simulink model "SkywalkerX8_Control"  (R2018a)
settings: Solver=FixedStepAuto  StartTime=0.0  StopTime=120  FixedStep=0.01  RelTol=1e-3
undefined symbols (not defined in the file): sigbuilder_block, SkywalkerX8
libraries: simulink x5, simulink_extras x3
(part 1 of 2)
settings Model: Creator=David  LastModifiedBy=David
settings OptimizationCC: DefaultParameterBehavior=Inlined  EnhancedBackFolding=on  PassReuseOutputArgsThreshold=0  OptimizeBlockOrder=speed  DifferentSizesBufferReuse=on  OptimizationCustomize=off
settings DebuggingCC: ParameterTunabilityLossMsg=error
settings SFSimCC: MATLABDynamicMemAlloc=off
settings RTWCC: GenCodeOnly=on  Description=Generic Real-Time Target  GenerateReport=on  LaunchReport=on
settings CodeAppCC: ForceParamTrailComments=on  OperatorAnnotations=on

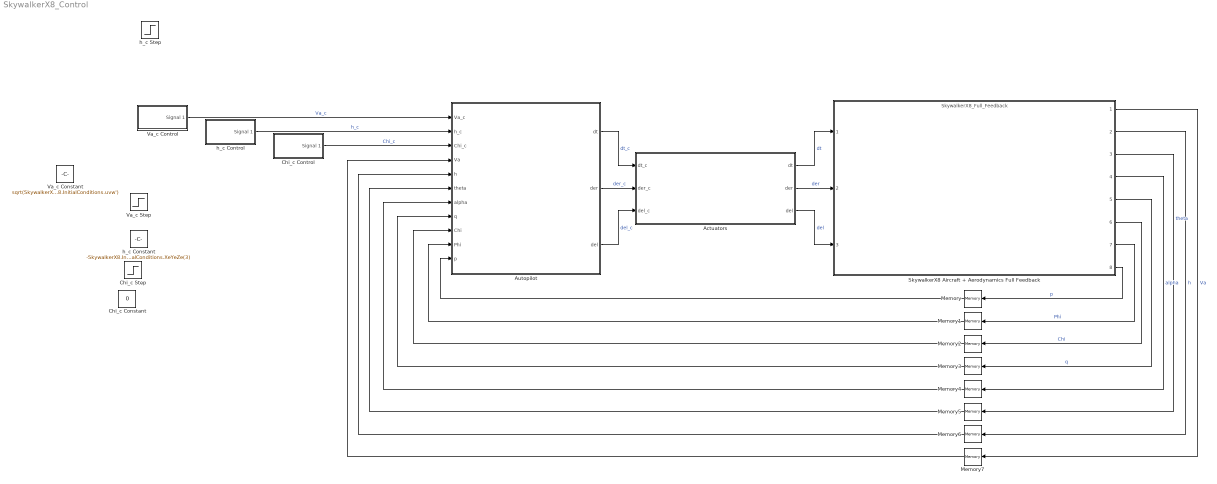
== system SkywalkerX8_Control ==
  Actuators : Subsystem
      mask Display:
      | image('actuators.jpg', 'center')
      | 
      | color('white')
      | 
      | port_label('input', 1, 'd_{t_c} (Unitless)', 'texmode', 'on')
      | port_label('input', 2, 'd_{{er}_c} (rad)', 'texmode', 'on')
      | port_label('input', 3, 'd_{{el}_c} (rad)', 'texmode', 'on')
      | 
      | port_label('output', 1, 'd_t (Unitless)', 'texmode', 'on')
      | port_label('output', 2, 'd_{er} (rad)', 'texmode', 'on')
      | port_label('output', 3, 'd_{el} (rad)', 'texmode', 'on')
  Autopilot : Subsystem
      mask Display:
      | image('autopilot.png', 'center')
      | 
      | port_label('output', 1, '\delta_t (Unitless)', 'texmode', 'on')
      | port_label('output', 2, '\delta_e_r (rad)', 'texmode', 'on')
      | port_label('output', 3, '\delta_e_l (rad)', 'texmode', 'on')
      | 
      | port_label('input', 1, 'V_{a_c} (m/s)', 'texmode', 'on')
      | port_label('input', 2, 'h_c (m)', 'texmode', 'on')
      | port_label('input', 3, '\chi_c (rad)', 'texmode', 'on')
      | port_label('input', 4, 'V_a (m/s)', 'texmode', 'on')
      | port_label('input', 5, 'Altitude (m)', 'texmode', 'on')
      | port_label('input', 6, '\theta (rad)', 'texmode', 'on')
      | port_label('input', 7, '\alpha (rad)', 'texmode', 'on')
      | port_label('input', 8, 'q (rad/s)', 'texmode', 'on')
      | port_label('input', 9, '\chi (rad)', 'texmode', 'on')
      | port_label('input', 10, '\phi (rad)', 'texmode', 'on')
      | port_label('input', 11, 'p (rad/s)', 'texmode', 'on')
  Chi_c Constant : Constant  Value=0
  Chi_c Control : Subsystem  Tag=STV Subsys  LoadFcn=sigbuilder_block('load');  StartFcn=sigbuilder_block('start');  StopFcn=sigbuilder_block('stop');  ClipboardFcn=sigbuilder_block('clipboard');  mask(Sigbuilder block){tuvar=[0:10]}
      mask help: Simulink:masks:SigbuilderBlock_MD
      mask init:
      | if ~strcmp(get_param(bdroot(gcbh),'SimulationStatus'),'stopped') tuvar = sigbuilder_block('maskInit'); end
      settings: CopyFcn=sigbuilder_block('copy');  DeleteFcn=sigbuilder_block('delete');  ModelCloseFcn=sigbuilder_block('modelClose');  PreSaveFcn=sigbuilder_block('preSave');  PauseFcn=sigbuilder_block('pause');  ContinueFcn=sigbuilder_block('continue');  NameChangeFcn=sigbuilder_block('namechange');  OpenFcn=sigbuilder_block('open',[437.6 199.2 550.4 400 ]);  CloseFcn=sigbuilder_block('close');
      mask Display: plot(0, 0, 100, 100,[2, 2, 32, 32, 2], [68, 8, 8, 68, 68],[32, 2], [38, 38], [32, 19, 2],[53, 60, 44], [32, 17, 17, 2],[16, 16, 31, 31]);txt = getActiveGroup(gcbh);text(2, 100, txt,'verticalAlignment', 'top');
  Chi_c Step : Step  After=deg2rad(90)  SampleTime=0
  Memory : Memory  InitialCondition=SkywalkerX8.InitialConditions.pqr(1)
  Memory1 : Memory  InitialCondition=SkywalkerX8.InitialConditions.PhiThetaPsi(1)
  Memory2 : Memory  InitialCondition=SkywalkerX8.InitialConditions.PhiThetaPsi(3)
  Memory3 : Memory  InitialCondition=SkywalkerX8.InitialConditions.pqr(2)
  Memory4 : Memory  InitialCondition=atan2(SkywalkerX8.InitialConditions.uvw(3), SkywalkerX8.InitialConditions.uvw(1))
  Memory5 : Memory  InitialCondition=SkywalkerX8.InitialConditions.PhiThetaPsi(2)
  Memory6 : Memory  InitialCondition=-SkywalkerX8.InitialConditions.XeYeZe(3)
  Memory7 : Memory  InitialCondition=sqrt(SkywalkerX8.InitialConditions.uvw*SkywalkerX8.InitialConditions.uvw')
  SkywalkerX8 Aircraft + Aerodynamics Full Feedback : ModelReference  ModelNameDialog=SkywalkerX8_Full_Feedback  ModelReferenceVersion=1.29
      mask Display:
      | image('x8SkySunset.png', 'center')
      | 
      | port_label('input', 1, '\delta_t (Unitless)', 'texmode', 'on')
      | port_label('input', 2, '\delta_e_r (rad)', 'texmode', 'on')
      | port_label('input', 3, '\delta_e_l (rad)', 'texmode', 'on')
      | 
      | port_label('output', 1, 'V_a (m/s)', 'texmode', 'on')
      | port_label('output', 2, 'Altitude (m)', 'texmode', 'on')
      | port_label('output', 3, '\theta (rad)', 'texmode', 'on')
      | port_label('output', 4, '\alpha (rad)', 'texmode', 'on')
      | port_label('output', 5, 'q (rad/s)', 'texmode', 'on')
      | port_label('output', 6, '\chi (rad)', 'texmode', 'on')
      | port_label('output', 7, '\phi (rad)', 'texmode', 'on')
      | port_label('output', 8, 'p (rad/s)', 'texmode', 'on')
  Va_c Constant : Constant  Value=sqrt(SkywalkerX8.InitialConditions.uvw*SkywalkerX8.InitialConditions.uvw')
  Va_c Control : Subsystem  Tag=STV Subsys  LoadFcn=sigbuilder_block('load');  StartFcn=sigbuilder_block('start');  StopFcn=sigbuilder_block('stop');  ClipboardFcn=sigbuilder_block('clipboard');  mask(Sigbuilder block){tuvar=[0:10]}
      mask help: Simulink:masks:SigbuilderBlock_MD
      mask init:
      | if ~strcmp(get_param(bdroot(gcbh),'SimulationStatus'),'stopped') tuvar = sigbuilder_block('maskInit'); end
      settings: CopyFcn=sigbuilder_block('copy');  DeleteFcn=sigbuilder_block('delete');  ModelCloseFcn=sigbuilder_block('modelClose');  PreSaveFcn=sigbuilder_block('preSave');  PauseFcn=sigbuilder_block('pause');  ContinueFcn=sigbuilder_block('continue');  NameChangeFcn=sigbuilder_block('namechange');  OpenFcn=sigbuilder_block('open',[437.6 199.2 550.4 400 ]);  CloseFcn=sigbuilder_block('close');
      mask Display: plot(0, 0, 100, 100,[2, 2, 32, 32, 2], [68, 8, 8, 68, 68],[32, 2], [38, 38], [32, 19, 2],[53, 60, 44], [32, 17, 17, 2],[16, 16, 31, 31]);txt = getActiveGroup(gcbh);text(2, 100, txt,'verticalAlignment', 'top');
  Va_c Step : Step  Before=sqrt(SkywalkerX8.InitialConditions.uvw*SkywalkerX8.InitialConditions.uvw')  After=sqrt(SkywalkerX8.InitialConditions.uvw*SkywalkerX8.InitialConditions.uvw')  SampleTime=0
  h_c Constant : Constant  Value=-SkywalkerX8.InitialConditions.XeYeZe(3)
  h_c Control : Subsystem  Tag=STV Subsys  LoadFcn=sigbuilder_block('load');  StartFcn=sigbuilder_block('start');  StopFcn=sigbuilder_block('stop');  ClipboardFcn=sigbuilder_block('clipboard');  mask(Sigbuilder block){tuvar=[0:10]}
      mask help: Simulink:masks:SigbuilderBlock_MD
      mask init:
      | if ~strcmp(get_param(bdroot(gcbh),'SimulationStatus'),'stopped') tuvar = sigbuilder_block('maskInit'); end
      settings: CopyFcn=sigbuilder_block('copy');  DeleteFcn=sigbuilder_block('delete');  ModelCloseFcn=sigbuilder_block('modelClose');  PreSaveFcn=sigbuilder_block('preSave');  PauseFcn=sigbuilder_block('pause');  ContinueFcn=sigbuilder_block('continue');  NameChangeFcn=sigbuilder_block('namechange');  OpenFcn=sigbuilder_block('open',[6 30 1428 771.75 ]);  CloseFcn=sigbuilder_block('close');
      mask Display: plot(0, 0, 100, 100,[2, 2, 32, 32, 2], [68, 8, 8, 68, 68],[32, 2], [38, 38], [32, 19, 2],[53, 60, 44], [32, 17, 17, 2],[16, 16, 31, 31]);txt = getActiveGroup(gcbh);text(2, 100, txt,'verticalAlignment', 'top');
  h_c Step : Step  Time=0.1  Before=-SkywalkerX8.InitialConditions.XeYeZe(3)  After=100  SampleTime=0
  wires:
  SkywalkerX8 Aircraft + Aerodynamics Full Feedback/6 -> Memory2/1  "Chi"
  SkywalkerX8 Aircraft + Aerodynamics Full Feedback/5 -> Memory3/1  "q"
  SkywalkerX8 Aircraft + Aerodynamics Full Feedback/4 -> Memory4/1  "alpha"
  SkywalkerX8 Aircraft + Aerodynamics Full Feedback/3 -> Memory5/1  "theta"
  SkywalkerX8 Aircraft + Aerodynamics Full Feedback/2 -> Memory6/1  "h"
  SkywalkerX8 Aircraft + Aerodynamics Full Feedback/1 -> Memory7/1  "Va"
  Memory/1 -> Autopilot/11(p)
  Memory1/1 -> Autopilot/10(Phi)
  Memory2/1 -> Autopilot/9(Chi)
  Memory3/1 -> Autopilot/8(q)
  Memory4/1 -> Autopilot/7(alpha)
  Memory5/1 -> Autopilot/6(theta)
  Memory6/1 -> Autopilot/5(h)
  Memory7/1 -> Autopilot/4(Va)
  h_c Control/1(Signal 1) -> Autopilot/2(h_c)  "h_c"
  Chi_c Control/1(Signal 1) -> Autopilot/3(Chi_c)  "Chi_c"
  Va_c Control/1(Signal 1) -> Autopilot/1(Va_c)  "Va_c"
  SkywalkerX8 Aircraft + Aerodynamics Full Feedback/8 -> Memory/1  "p"
  SkywalkerX8 Aircraft + Aerodynamics Full Feedback/7 -> Memory1/1  "Phi"
  Autopilot/1(dt) -> Actuators/1(dt_c)  "dt_c"
  Actuators/1(dt) -> SkywalkerX8 Aircraft + Aerodynamics Full Feedback/1  "dt"
  Autopilot/2(der) -> Actuators/2(der_c)  "der_c"
  Actuators/2(der) -> SkywalkerX8 Aircraft + Aerodynamics Full Feedback/2  "der"
  Autopilot/3(del) -> Actuators/3(del_c)  "del_c"
  Actuators/3(del) -> SkywalkerX8 Aircraft + Aerodynamics Full Feedback/3  "del"

== system SkywalkerX8_Control/Actuators ==
  dt_c : Inport
  der_c : Inport  Port=2
  del_c : Inport  Port=3
  Left Servo-Motor : Subsystem
      mask Display: image('servo.jpg', 'center')
  Motor Model : simulink_extras/Additional Linear/State-Space (with initial outputs)  A=SkywalkerX8.Actuators.Motor.SS.A  B=SkywalkerX8.Actuators.Motor.SS.B  C=SkywalkerX8.Actuators.Motor.SS.C  D=SkywalkerX8.Actuators.Motor.SS.D  U0=SkywalkerX8.InitialConditions.dt  Y0=SkywalkerX8.InitialConditions.dt  mask(State-Space with Initial Outputs){}
      settings: SourceProductName=Simulink  SourceProductBaseCode=SL
      mask Display: image('motor.jpg', 'center')
  Right Servo-Motor : Subsystem
      mask Display: image('servo.jpg', 'center')
  dt : Outport
  der : Outport  Port=2
  del : Outport  Port=3
  wires:
  del_c/1 -> Left Servo-Motor/1(del_c)
  Motor Model/1 -> dt/1
  Left Servo-Motor/1(del) -> del/1
  der_c/1 -> Right Servo-Motor/1(der_c)
  dt_c/1 -> Motor Model/1
  Right Servo-Motor/1(der) -> der/1

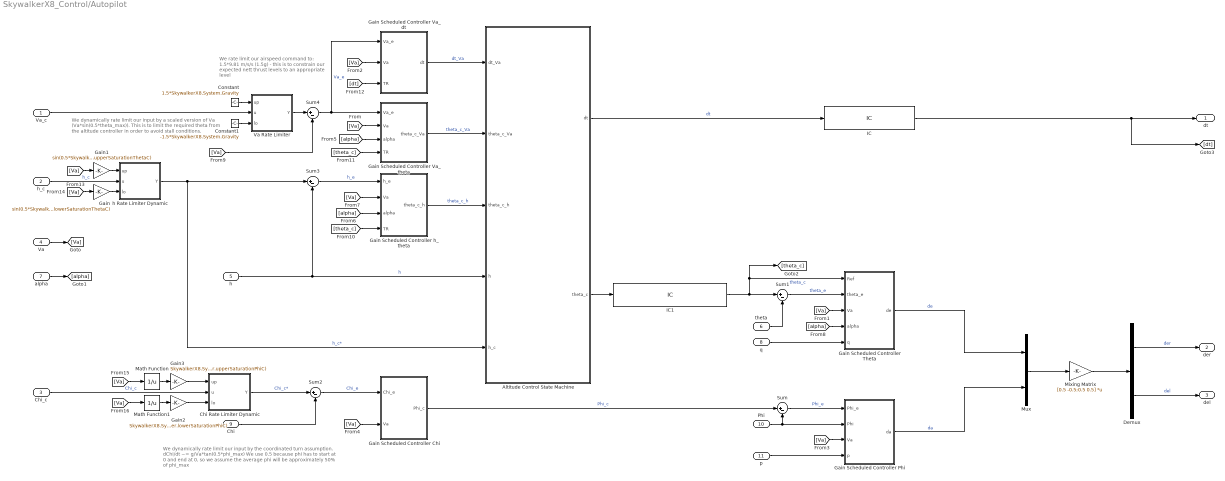
== system SkywalkerX8_Control/Autopilot ==
  note: We dynamically rate limit our input
      | by a scaled version of Va (Va*sin(0.5*theta_max)).
      |
      | This is to limit the required theta from the altitude controller
      | in order to avoid stall conditions.
  note: We dynamically rate limit our input
      | by the coordinated turn assumption.
      |
      | dChi/dt ~= g/Va*tan(0.5*phi_max)
      |
      | We use 0.5 because phi has to start at 0 and end at 0, so we assume
      | the average phi will be approximately 50% of phi_max
  note: We rate limit our airspeed command to:
      |
      | 1.5*9.81 m/s/s (1.5g) - this is to constrain our expected nett thrust levels to an appropriate level
  Va_c : Inport
  h_c : Inport  Port=2
  Chi_c : Inport  Port=3
  Va : Inport  Port=4
  h : Inport  Port=5
  theta : Inport  Port=6
  alpha : Inport  Port=7
  q : Inport  Port=8
  Chi : Inport  Port=9
  Phi : Inport  Port=10
  p : Inport  Port=11
  Altitude Control State Machine : Stateflow chart  TreatAsAtomicUnit=on  mask{h_hold=SkywalkerX8.Control.Longitudinal.AltStateMachine.hHold, h_takeoff=SkywalkerX8.Control.Longitudinal.AltStateMachine.hTakeOff, theta_c_takeoff=SkywalkerX8.Control.Longitudinal.AltStateMachine.thetaTakeOff, hyst_frac=SkywalkerX8.Control.Longitudinal.AltStateMachine.HysteresisFraction, PreFlightBypass=SkywalkerX8.Control.Longitudinal.AltStateMachine.PreFlightBypass}
      mask prompts: h_hold "Altitude hold zone (+- band around the commanded altitude where theta will control altitude) (m)"; h_takeoff "Takeoff altitude (altitude after which we move away from constant pitch angle command) (m)"; theta_c_takeoff "Takeoff pitch angle (constant pitch angle at which to climb at at takeoff) (rad)"; hyst_frac "Hysteresis Fraction (Unitless)"; PreFlightBypass "Preflight Bypass (Unitless)"
  Chi Rate Limiter Dynamic : Subsystem  mask{initOutput=SkywalkerX8.InitialConditions.PhiThetaPsi(3)}
      mask prompts: initOutput "Initial output of dynamic rate limiter"
      mask DialogControl DescGroupVar Prompt: Rate Limiter Dynamic
      mask DialogControl DescTextVar Prompt: Limit rising and falling rates of the signals at the second input by using the first input (upper limit) and the third input (lower limit).
      mask Display:
      | image('rateLimit.png')
      | 
      | port_label('input', 1, 'up')
      | port_label('input', 2, 'u')
      | port_label('input', 3, 'lo')
      | 
      | port_label('output', 1, 'Y')
  Constant : Constant  Value=1.5*SkywalkerX8.System.Gravity
  Constant1 : Constant  Value=-1.5*SkywalkerX8.System.Gravity
  Demux : Demux  Outputs=2
  Gain : Gain  Gain=sin(0.5*SkywalkerX8.Control.Longitudinal.altController.lowerSaturationThetaC)
  Gain Scheduled Controller Chi : Subsystem
  Gain Scheduled Controller Phi : Subsystem
  Gain Scheduled Controller Theta : Subsystem
  Gain Scheduled Controller Va_dt : Subsystem
  Gain Scheduled Controller Va_theta : Subsystem
  Gain Scheduled Controller h_theta : Subsystem
  Gain1 : Gain  Gain=sin(0.5*SkywalkerX8.Control.Longitudinal.altController.upperSaturationThetaC)
  Gain2 : Gain  Gain=SkywalkerX8.System.Gravity*tan(0.5*SkywalkerX8.Control.Lateral.ChiController.lowerSaturationPhiC)
  Gain3 : Gain  Gain=SkywalkerX8.System.Gravity*tan(0.5*SkywalkerX8.Control.Lateral.ChiController.upperSaturationPhiC)
  IC : InitialCondition  Value=SkywalkerX8.InitialConditions.dt
  IC1 : InitialCondition  Value=SkywalkerX8.InitialConditions.PhiThetaPsi(2)
  Math Function : Math  Operator=reciprocal  SaturateOnIntegerOverflow=on
  Math Function1 : Math  Operator=reciprocal  SaturateOnIntegerOverflow=on
  Mixing Matrix : Gain  Gain=[0.5 -0.5;0.5 0.5]  Multiplication=Matrix(K*u)
  Mux : Mux  Inputs=2
  Sum{,1..4} (5 alike) : Sum  Inputs=|+-
  Va Rate Limiter : Subsystem  mask{initOutput=sqrt(SkywalkerX8.InitialConditions.uvw*SkywalkerX8.InitialConditions.uvw')}
      mask prompts: initOutput "Initial output of dynamic rate limiter"
      mask DialogControl DescGroupVar Prompt: Rate Limiter Dynamic
      mask DialogControl DescTextVar Prompt: Limit rising and falling rates of the signals at the second input by using the first input (upper limit) and the third input (lower limit).
      mask Display:
      | image('rateLimit.png')
      | 
      | port_label('input', 1, 'up')
      | port_label('input', 2, 'u')
      | port_label('input', 3, 'lo')
      | 
      | port_label('output', 1, 'Y')
  h Rate Limiter Dynamic : Subsystem  mask{initOutput=-SkywalkerX8.InitialConditions.XeYeZe(3)}
      mask prompts: initOutput "Initial output of dynamic rate limiter"
      mask DialogControl DescGroupVar Prompt: Rate Limiter Dynamic
      mask DialogControl DescTextVar Prompt: Limit rising and falling rates of the signals at the second input by using the first input (upper limit) and the third input (lower limit).
      mask Display:
      | image('rateLimit.png')
      | 
      | port_label('input', 1, 'up')
      | port_label('input', 2, 'u')
      | port_label('input', 3, 'lo')
      | 
      | port_label('output', 1, 'Y')
  dt : Outport
  der : Outport  Port=2
  del : Outport  Port=3
  wires:
  [Va] -> Sum4/2
  Sum4/1 -> Gain Scheduled Controller Va_theta/1(Va_e), Gain Scheduled Controller Va_dt/1(Va_e)  "Va_e"
  Demux/1 -> der/1  "der"
  Gain Scheduled Controller Chi/1(Phi_c) -> Sum/1  "Phi_c"
  h/1 -> Altitude Control State Machine/4(h), Sum3/2  "h"
  h Rate Limiter Dynamic/1(Y) -> Altitude Control State Machine/5(h_c), Sum3/1  "h_c*"
  Chi Rate Limiter Dynamic/1(Y) -> Sum2/1  "Chi_c*"
  Sum3/1 -> Gain Scheduled Controller h_theta/1(h_e)  "h_e"
  Sum2/1 -> Gain Scheduled Controller Chi/1(Chi_e)  "Chi_e"
  Phi/1 -> Gain Scheduled Controller Phi/2(Phi), Sum/2
  Sum/1 -> Gain Scheduled Controller Phi/1(Phi_e)  "Phi_e"
  Gain Scheduled Controller Phi/1(da) -> Mux/2  "da"
  [Va] -> Gain Scheduled Controller Phi/3(Va)
  [Va] -> Gain Scheduled Controller Theta/3(Va)
  Va_c/1 -> Va Rate Limiter/2(u)
  [alpha] -> Gain Scheduled Controller Va_theta/3(alpha)
  [Va] -> Gain Scheduled Controller Chi/2(Va)
  Sum1/1 -> Gain Scheduled Controller Theta/2(theta_e)  "theta_e"
  [Va] -> Gain Scheduled Controller Va_dt/2(Va)
  Demux/2 -> del/1  "del"
  alpha/1 -> [alpha]
  [Va] -> Gain Scheduled Controller Va_theta/2(Va)
  Chi/1 -> Sum2/2
  Gain Scheduled Controller Theta/1(de) -> Mux/1  "de"
  p/1 -> Gain Scheduled Controller Phi/4(p)
  Va/1 -> [Va]
  theta/1 -> Sum1/2
  Mux/1 -> Mixing Matrix/1
  Mixing Matrix/1 -> Demux/1
  [Va] -> Gain Scheduled Controller h_theta/2(Va)
  [alpha] -> Gain Scheduled Controller h_theta/3(alpha)
  Altitude Control State Machine/1(dt) -> IC/1  "dt"
  Gain Scheduled Controller Va_theta/1(theta_c_Va) -> Altitude Control State Machine/2(theta_c_Va)  "theta_c_Va"
  [theta_c] -> Gain Scheduled Controller Va_theta/4(TR)
  [dt] -> Gain Scheduled Controller Va_dt/3(TR)
  IC/1 -> dt/1, [dt]
  [theta_c] -> Gain Scheduled Controller h_theta/4(TR)
  IC1/1 -> Gain Scheduled Controller Theta/1(Ref), [theta_c], Sum1/1  "theta_c"
  [alpha] -> Gain Scheduled Controller Theta/4(alpha)
  q/1 -> Gain Scheduled Controller Theta/5(q)
  Gain Scheduled Controller h_theta/1(theta_c_h) -> Altitude Control State Machine/3(theta_c_h)  "theta_c_h"
  Altitude Control State Machine/2(theta_c) -> IC1/1
  Gain Scheduled Controller Va_dt/1(dt) -> Altitude Control State Machine/1(dt_Va)  "dt_Va"
  h_c/1 -> h Rate Limiter Dynamic/2(u)  "h_c"
  [Va] -> Gain1/1
  Gain/1 -> h Rate Limiter Dynamic/3(lo)
  [Va] -> Gain/1
  Gain1/1 -> h Rate Limiter Dynamic/1(up)
  [Va] -> Math Function1/1
  [Va] -> Math Function/1
  Gain2/1 -> Chi Rate Limiter Dynamic/3(lo)
  Gain3/1 -> Chi Rate Limiter Dynamic/1(up)
  Chi_c/1 -> Chi Rate Limiter Dynamic/2(u)  "Chi_c"
  Math Function/1 -> Gain3/1
  Math Function1/1 -> Gain2/1
  Va Rate Limiter/1(Y) -> Sum4/1
  Constant/1 -> Va Rate Limiter/1(up)
  Constant1/1 -> Va Rate Limiter/3(lo)

== system SkywalkerX8_Control/Chi_c Control ==
  Demux : Demux  Tag=STV Demux  Outputs=1
  FromWs : FromWorkspace  Tag=STV FromWs  VariableName=tuvar  SampleTime=0
      SigBuilderData=|
      | common.afterFinalStr = 'Extrapolate'
      | common.sampleTime = 0
      | dataSet.timeRange = [0 120]
      | dataSet.name = 'Group 1'
      | sbobj.Groups.Name = 'Group 1'
      | sbobj.Groups.Signals.Name = 'Signal 1'
      | sbobj.Groups.Signals.XData = [0 10 10 35 35 55 55 90 90 120]
      | sbobj.Groups.Signals.YData = [0 0 1.5708 1.5708 0 0 1.5708 1.5708 0 0]
      | sbobj.Groups.TimeRange = [0 120]
  Signal 1 : Outport  Tag=STV Outport
  wires:
  Demux/1 -> Signal 1/1
  FromWs/1 -> Demux/1

== system SkywalkerX8_Control/Va_c Control ==
  Demux : Demux  Tag=STV Demux  Outputs=1
  FromWs : FromWorkspace  Tag=STV FromWs  VariableName=tuvar  SampleTime=0
      SigBuilderData=|
      | common.afterFinalStr = 'Extrapolate'
      | common.sampleTime = 0
      | dataSet.timeRange = [0 120]
      | dataSet.name = 'Group 1'
      | sbobj.Groups.Name = 'Group 1'
      | sbobj.Groups.Signals.Name = 'Signal 1'
      | sbobj.Groups.Signals.XData = [0 10 10 30 30 50 50 70 70 120]
      | sbobj.Groups.Signals.YData = [17.3072 17.3 20 20 17.3072 17.3072 15 15 17.3072 17.3072]
      | sbobj.Groups.TimeRange = [0 120]
  Signal 1 : Outport  Tag=STV Outport
  wires:
  Demux/1 -> Signal 1/1
  FromWs/1 -> Demux/1

== system SkywalkerX8_Control/h_c Control ==
  Demux : Demux  Tag=STV Demux  Outputs=1
  FromWs : FromWorkspace  Tag=STV FromWs  VariableName=tuvar  SampleTime=0
      SigBuilderData=|
      | common.afterFinalStr = 'Extrapolate'
      | common.sampleTime = 0
      | dataSet.timeRange = [0 120]
      | dataSet.name = 'Group 1'
      | sbobj.Groups.Name = 'Group 1'
      | sbobj.Groups.Signals.Name = 'Signal 1'
      | sbobj.Groups.Signals.XData = [0 1 1 20 20 40 40 60 80 80 100 100 120]
      | sbobj.Groups.Signals.YData = [50 50 60 60 75 75 100 100 80 60 60 100 100]
      | sbobj.Groups.TimeRange = [0 120]
  Signal 1 : Outport  Tag=STV Outport
  wires:
  Demux/1 -> Signal 1/1
  FromWs/1 -> Demux/1

== system SkywalkerX8_Control/Actuators/Left Servo-Motor ==
  del_c : Inport
  Abs : Abs
  Compare To Constant : simulink/Logic and Bit Operations/Compare To Constant  relop=>  const=SkywalkerX8.Actuators.Servos.RateLimit  OutDataTypeStr=boolean
  Derivative : Derivative
  Rate Limiter : RateLimiter  Commented=through  RisingSlewLimit=SkywalkerX8.Actuators.Servos.RateLimit  FallingSlewLimit=-SkywalkerX8.Actuators.Servos.RateLimit  SampleTimeMode=inherited  InitialCondition=SkywalkerX8.InitialConditions.de*0.5 + SkywalkerX8.InitialConditions.da*0.5
  Saturation : Saturate  UpperLimit=SkywalkerX8.Actuators.Servos.UpperSaturation  LowerLimit=SkywalkerX8.Actuators.Servos.LowerSaturation
  Second Order Servo-Motor Model : simulink_extras/Additional Linear/State-Space (with initial outputs)  A=SkywalkerX8.Actuators.Servos.SS.A  B=SkywalkerX8.Actuators.Servos.SS.B  C=SkywalkerX8.Actuators.Servos.SS.C  D=SkywalkerX8.Actuators.Servos.SS.D  U0=(SkywalkerX8.InitialConditions.de*0.5 + SkywalkerX8.InitialConditions.da*0.5)  Y0=(SkywalkerX8.InitialConditions.de*0.5 + SkywalkerX8.InitialConditions.da*0.5)
      settings: SourceProductName=Simulink  SourceProductBaseCode=SL
  Terminator : Terminator
  del : Outport
  wires:
  Rate Limiter/1 -> Saturation/1
  del_c/1 -> Second Order Servo-Motor Model/1
  Saturation/1 -> del/1
  Derivative/1 -> Abs/1
  Abs/1 -> Compare To Constant/1
  Compare To Constant/1 -> Terminator/1  "lServoRateLimitCheck"
  Second Order Servo-Motor Model/1 -> Derivative/1, Rate Limiter/1

== system SkywalkerX8_Control/Actuators/Right Servo-Motor ==
  der_c : Inport
  Abs : Abs
  Compare To Constant : simulink/Logic and Bit Operations/Compare To Constant  relop=>  const=SkywalkerX8.Actuators.Servos.RateLimit  OutDataTypeStr=boolean
  Derivative : Derivative
  Rate Limiter : RateLimiter  Commented=through  RisingSlewLimit=SkywalkerX8.Actuators.Servos.RateLimit  FallingSlewLimit=-SkywalkerX8.Actuators.Servos.RateLimit  SampleTimeMode=inherited  InitialCondition=SkywalkerX8.InitialConditions.de*0.5 - SkywalkerX8.InitialConditions.da*0.5
  Saturation : Saturate  UpperLimit=SkywalkerX8.Actuators.Servos.UpperSaturation  LowerLimit=SkywalkerX8.Actuators.Servos.LowerSaturation
  Second Order Servo-Motor Model : simulink_extras/Additional Linear/State-Space (with initial outputs)  A=SkywalkerX8.Actuators.Servos.SS.A  B=SkywalkerX8.Actuators.Servos.SS.B  C=SkywalkerX8.Actuators.Servos.SS.C  D=SkywalkerX8.Actuators.Servos.SS.D  U0=(SkywalkerX8.InitialConditions.de*0.5 - SkywalkerX8.InitialConditions.da*0.5)  Y0=(SkywalkerX8.InitialConditions.de*0.5 - SkywalkerX8.InitialConditions.da*0.5)
      settings: SourceProductName=Simulink  SourceProductBaseCode=SL
  Terminator : Terminator
  der : Outport
  wires:
  Rate Limiter/1 -> Saturation/1
  der_c/1 -> Second Order Servo-Motor Model/1
  Second Order Servo-Motor Model/1 -> Derivative/1, Rate Limiter/1
  Saturation/1 -> der/1
  Derivative/1 -> Abs/1
  Abs/1 -> Compare To Constant/1
  Compare To Constant/1 -> Terminator/1  "rServoRateLimitCheck"

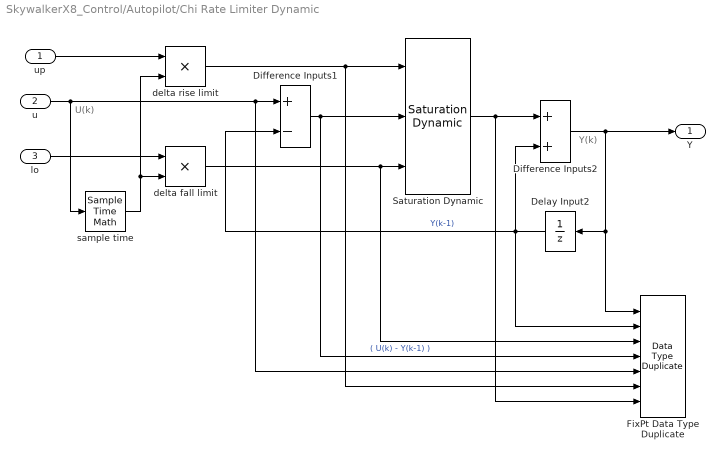
== system SkywalkerX8_Control/Autopilot/Chi Rate Limiter Dynamic ==
  note: U(k)
  note: Y(k)
  up : Inport
  u : Inport  Port=2
  lo : Inport  Port=3
  Delay Input2 : UnitDelay  Description=Store in Global RAM  DisableCoverage=on  InitialCondition=initOutput  SampleTime=-1
  Difference Inputs1 : Sum  Description=Add in CPU  DisableCoverage=on  Inputs=+-  OutDataTypeStr=Inherit: Inherit via back propagation
  Difference Inputs2 : Sum  Description=Add in CPU  OutDataTypeStr=Inherit: Inherit via back propagation
  FixPt Data Type Duplicate : DataTypeDuplicate  DisableCoverage=on  NumInputPorts=7
  Saturation Dynamic : simulink/Discontinuities/Saturation Dynamic  OutMin=[]  OutMax=[]  OutDataTypeStr=Inherit: Same as second input  OutDataType=fixdt(1, 16)  OutScaling=2^-10  DoSatur=off
  delta fall limit : Product  DisableCoverage=on  Inputs=**  OutDataTypeStr=Inherit: Inherit via back propagation  SaturateOnIntegerOverflow=on
  delta rise limit : Product  DisableCoverage=on  Inputs=**  OutDataTypeStr=Inherit: Inherit via back propagation  SaturateOnIntegerOverflow=on
  sample time : SampleTimeMath  DisableCoverage=on  TsampMathOp=Ts Only  weightValue=1
  Y : Outport  InitialOutput=0
  wires:
  Delay Input2/1 -> Difference Inputs1/2, FixPt Data Type Duplicate/2, Difference Inputs2/2  "Y(k-1)"
  Difference Inputs1/1 -> FixPt Data Type Duplicate/4, Saturation Dynamic/2  "( U(k) - Y(k-1) )"
  Difference Inputs2/1 -> Y/1, Delay Input2/1, FixPt Data Type Duplicate/1
  u/1 -> Difference Inputs1/1, FixPt Data Type Duplicate/5, sample time/1
  delta fall limit/1 -> FixPt Data Type Duplicate/3, Saturation Dynamic/3
  sample time/1 -> delta fall limit/2, delta rise limit/2
  Saturation Dynamic/1 -> Difference Inputs2/1, FixPt Data Type Duplicate/7
  delta rise limit/1 -> FixPt Data Type Duplicate/6, Saturation Dynamic/1
  lo/1 -> delta fall limit/1
  up/1 -> delta rise limit/1

== system SkywalkerX8_Control/Autopilot/Gain Scheduled Controller Chi ==
  Chi_e : Inport
  Va : Inport  Port=2
  PIDF Controller Chi Kd 2D Lookup Table : Lookup_n-D  NumberOfTableDimensions=1  BreakpointsForDimension1=SkywalkerX8.Control.Lateral.SchedulingVariables.VaArray  BreakpointsForDimension2=SkywalkerX8.Control.Longitudinal.SchedulingVariables.alphaArray  Table=SkywalkerX8.Control.Lateral.ChiController.KdChi  InternalRulePriority=Speed  RndMeth=Simplest  InputSameDT=on
  PIDF Controller Chi Ki 2D Lookup Table : Lookup_n-D  NumberOfTableDimensions=1  BreakpointsForDimension1=SkywalkerX8.Control.Lateral.SchedulingVariables.VaArray  BreakpointsForDimension2=SkywalkerX8.Control.Longitudinal.SchedulingVariables.alphaArray  Table=SkywalkerX8.Control.Lateral.ChiController.KiChi  InternalRulePriority=Speed  RndMeth=Simplest  InputSameDT=on
  PIDF Controller Chi Kp 2D Lookup Table : Lookup_n-D  NumberOfTableDimensions=1  BreakpointsForDimension1=SkywalkerX8.Control.Lateral.SchedulingVariables.VaArray  BreakpointsForDimension2=SkywalkerX8.Control.Longitudinal.SchedulingVariables.alphaArray  Table=SkywalkerX8.Control.Lateral.ChiController.KpChi  InternalRulePriority=Speed  RndMeth=Simplest  InputSameDT=on
  PIDF Controller Chi N 2D Lookup Table : Lookup_n-D  NumberOfTableDimensions=1  BreakpointsForDimension1=SkywalkerX8.Control.Lateral.SchedulingVariables.VaArray  BreakpointsForDimension2=SkywalkerX8.Control.Longitudinal.SchedulingVariables.alphaArray  Table=SkywalkerX8.Control.Lateral.ChiController.NChi  InternalRulePriority=Speed  RndMeth=Simplest  InputSameDT=on
  PIDF Controller Va_theta : Subsystem
  Saturation : Saturate  UpperLimit=SkywalkerX8.Control.Lateral.ChiController.upperSaturationPhiC  LowerLimit=SkywalkerX8.Control.Lateral.ChiController.lowerSaturationPhiC
  Phi_c : Outport
  wires:
  PIDF Controller Chi Kp 2D Lookup Table/1 -> PIDF Controller Va_theta/2(P)
  Chi_e/1 -> PIDF Controller Va_theta/1(u)
  Va/1 -> PIDF Controller Chi Kp 2D Lookup Table/1, PIDF Controller Chi Ki 2D Lookup Table/1, PIDF Controller Chi N 2D Lookup Table/1, PIDF Controller Chi Kd 2D Lookup Table/1
  PIDF Controller Chi Ki 2D Lookup Table/1 -> PIDF Controller Va_theta/3(I)
  PIDF Controller Chi Kd 2D Lookup Table/1 -> PIDF Controller Va_theta/4(D)
  PIDF Controller Chi N 2D Lookup Table/1 -> PIDF Controller Va_theta/5(N)
  Saturation/1 -> PIDF Controller Va_theta/6(Post-Saturation), Phi_c/1
  PIDF Controller Va_theta/1(y) -> PIDF Controller Va_theta/7(Pre-Saturation), Saturation/1

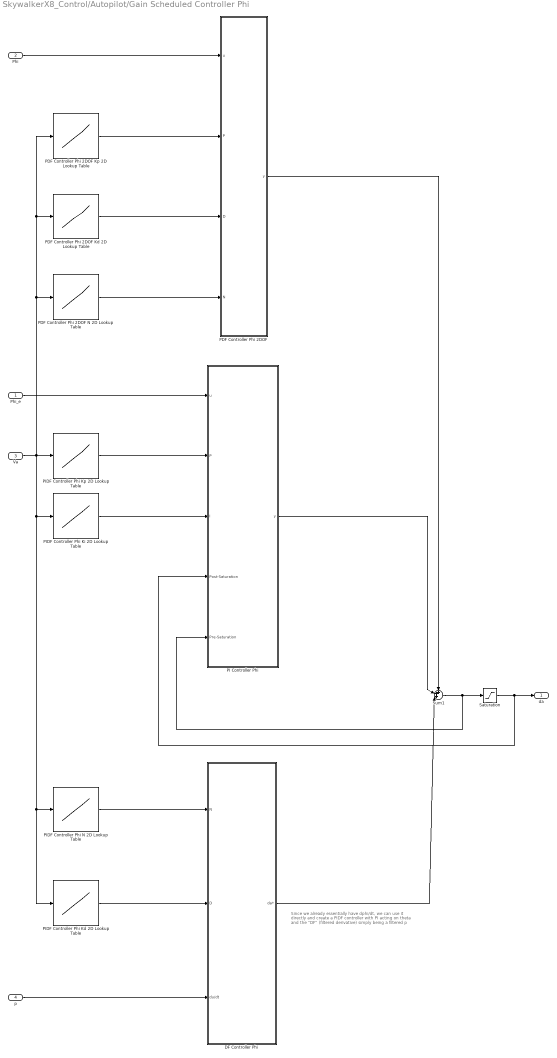
== system SkywalkerX8_Control/Autopilot/Gain Scheduled Controller Phi ==
  note: Since we already essentially have dphi/dt,
      | we can use it directly and create a PIDF controller
      | with PI acting on theta and the "DF" (filtered derivative)
      | simply being a filtered p
  Phi_e : Inport
  Phi : Inport  Port=2
  Va : Inport  Port=3
  p : Inport  Port=4
  DF Controller Phi : Subsystem
  PDF Controller Phi 2DOF : Subsystem
  PDF Controller Phi 2DOF Kd 2D Lookup Table : Lookup_n-D  NumberOfTableDimensions=1  BreakpointsForDimension1=SkywalkerX8.Control.Lateral.SchedulingVariables.VaArray  BreakpointsForDimension2=SkywalkerX8.Control.Longitudinal.SchedulingVariables.alphaArray  Table=SkywalkerX8.Control.Lateral.PhiController.KdPhi2DOF  InternalRulePriority=Speed  RndMeth=Simplest  InputSameDT=on
  PDF Controller Phi 2DOF Kp 2D Lookup Table : Lookup_n-D  NumberOfTableDimensions=1  BreakpointsForDimension1=SkywalkerX8.Control.Lateral.SchedulingVariables.VaArray  BreakpointsForDimension2=SkywalkerX8.Control.Longitudinal.SchedulingVariables.alphaArray  Table=SkywalkerX8.Control.Lateral.PhiController.KpPhi2DOF  InternalRulePriority=Speed  RndMeth=Simplest  InputSameDT=on
  PDF Controller Phi 2DOF N 2D Lookup Table : Lookup_n-D  NumberOfTableDimensions=1  BreakpointsForDimension1=SkywalkerX8.Control.Lateral.SchedulingVariables.VaArray  BreakpointsForDimension2=SkywalkerX8.Control.Longitudinal.SchedulingVariables.alphaArray  Table=SkywalkerX8.Control.Lateral.PhiController.NPhi2DOF  InternalRulePriority=Speed  RndMeth=Simplest  InputSameDT=on
  PI Controller Phi : Subsystem
  PIDF Controller Phi Kd 2D Lookup Table : Lookup_n-D  NumberOfTableDimensions=1  BreakpointsForDimension1=SkywalkerX8.Control.Lateral.SchedulingVariables.VaArray  BreakpointsForDimension2=SkywalkerX8.Control.Longitudinal.SchedulingVariables.alphaArray  Table=SkywalkerX8.Control.Lateral.PhiController.KdPhi  InternalRulePriority=Speed  RndMeth=Simplest  InputSameDT=on
  PIDF Controller Phi Ki 2D Lookup Table : Lookup_n-D  NumberOfTableDimensions=1  BreakpointsForDimension1=SkywalkerX8.Control.Lateral.SchedulingVariables.VaArray  BreakpointsForDimension2=SkywalkerX8.Control.Longitudinal.SchedulingVariables.alphaArray  Table=SkywalkerX8.Control.Lateral.PhiController.KiPhi  InternalRulePriority=Speed  RndMeth=Simplest  InputSameDT=on
  PIDF Controller Phi Kp 2D Lookup Table : Lookup_n-D  NumberOfTableDimensions=1  BreakpointsForDimension1=SkywalkerX8.Control.Lateral.SchedulingVariables.VaArray  BreakpointsForDimension2=SkywalkerX8.Control.Longitudinal.SchedulingVariables.alphaArray  Table=SkywalkerX8.Control.Lateral.PhiController.KpPhi  InternalRulePriority=Speed  RndMeth=Simplest  InputSameDT=on
  PIDF Controller Phi N 2D Lookup Table : Lookup_n-D  NumberOfTableDimensions=1  BreakpointsForDimension1=SkywalkerX8.Control.Lateral.SchedulingVariables.VaArray  BreakpointsForDimension2=SkywalkerX8.Control.Longitudinal.SchedulingVariables.alphaArray  Table=SkywalkerX8.Control.Lateral.PhiController.NPhi  InternalRulePriority=Speed  RndMeth=Simplest  InputSameDT=on
  Saturation : Saturate  UpperLimit=SkywalkerX8.Control.Lateral.PhiController.upperSaturationDa  LowerLimit=SkywalkerX8.Control.Lateral.PhiController.lowerSaturationDa
  Sum1 : Sum  Inputs=+++|
  da : Outport
  wires:
  Va/1 -> PDF Controller Phi 2DOF Kp 2D Lookup Table/1, PDF Controller Phi 2DOF Kd 2D Lookup Table/1, PDF Controller Phi 2DOF N 2D Lookup Table/1, PIDF Controller Phi N 2D Lookup Table/1, PIDF Controller Phi Kd 2D Lookup Table/1, PIDF Controller Phi Ki 2D Lookup Table/1, PIDF Controller Phi Kp 2D Lookup Table/1
  Phi_e/1 -> PI Controller Phi/1(u)
  PIDF Controller Phi Kp 2D Lookup Table/1 -> PI Controller Phi/2(P)
  PIDF Controller Phi Ki 2D Lookup Table/1 -> PI Controller Phi/3(I)
  PI Controller Phi/1(y) -> Sum1/2
  Sum1/1 -> Saturation/1, PI Controller Phi/5(Pre-Saturation)
  p/1 -> DF Controller Phi/3(du/dt)
  DF Controller Phi/1(da*) -> Sum1/3
  PIDF Controller Phi N 2D Lookup Table/1 -> DF Controller Phi/1(N)
  PIDF Controller Phi Kd 2D Lookup Table/1 -> DF Controller Phi/2(D)
  Saturation/1 -> da/1, PI Controller Phi/4(Post-Saturation)
  PDF Controller Phi 2DOF Kp 2D Lookup Table/1 -> PDF Controller Phi 2DOF/2(P)
  PDF Controller Phi 2DOF Kd 2D Lookup Table/1 -> PDF Controller Phi 2DOF/3(D)
  PDF Controller Phi 2DOF N 2D Lookup Table/1 -> PDF Controller Phi 2DOF/4(N)
  Phi/1 -> PDF Controller Phi 2DOF/1(u)
  PDF Controller Phi 2DOF/1(y) -> Sum1/1

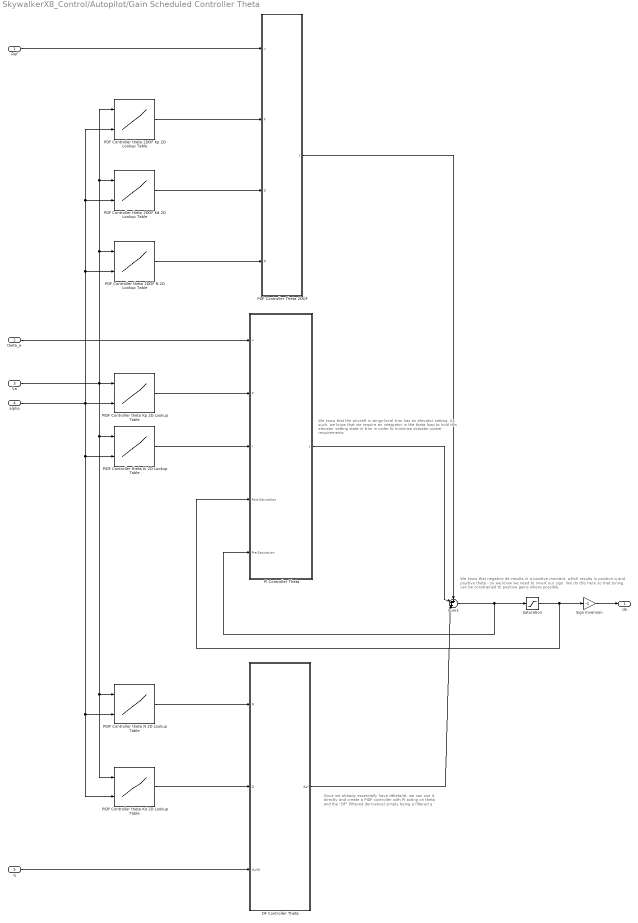
== system SkywalkerX8_Control/Autopilot/Gain Scheduled Controller Theta ==
  note: Since we already essentially have dtheta/dt,
      | we can use it directly and create a PIDF controller
      | with PI acting on theta and the "DF" (filtered derivative)
      | simply being a filtered q
  note: We know that negative de results in a positive moment, which results in
      | positive q and positive theta - so we know we need to invert our sign.
      | We do this here so that tuning can be constrained to positive gains where possible.
  note: We know that the aircraft in wings-level trim has an elevator setting. As such, we know that we require an integrator in the theta loop to hold this elevator setting state in trim in order to minimize actuator power requirements.
  Ref : Inport
  theta_e : Inport  Port=2
  Va : Inport  Port=3
  alpha : Inport  Port=4
  q : Inport  Port=5
  DF Controller Theta : Subsystem
  PDF Controller Theta 2DOF : Subsystem
  PDF Controller theta 2DOF Kd 2D Lookup Table : Lookup_n-D  BreakpointsForDimension1=SkywalkerX8.Control.Longitudinal.SchedulingVariables.VaArray  BreakpointsForDimension2=SkywalkerX8.Control.Longitudinal.SchedulingVariables.alphaArray  Table=SkywalkerX8.Control.Longitudinal.thetaController.KdTheta2DOF  InternalRulePriority=Speed  RndMeth=Simplest  InputSameDT=on
  PDF Controller theta 2DOF Kp 2D Lookup Table : Lookup_n-D  BreakpointsForDimension1=SkywalkerX8.Control.Longitudinal.SchedulingVariables.VaArray  BreakpointsForDimension2=SkywalkerX8.Control.Longitudinal.SchedulingVariables.alphaArray  Table=SkywalkerX8.Control.Longitudinal.thetaController.KpTheta2DOF  InternalRulePriority=Speed  RndMeth=Simplest  InputSameDT=on
  PDF Controller theta 2DOF N 2D Lookup Table : Lookup_n-D  BreakpointsForDimension1=SkywalkerX8.Control.Longitudinal.SchedulingVariables.VaArray  BreakpointsForDimension2=SkywalkerX8.Control.Longitudinal.SchedulingVariables.alphaArray  Table=SkywalkerX8.Control.Longitudinal.thetaController.NTheta2DOF  InternalRulePriority=Speed  RndMeth=Simplest  InputSameDT=on
  PI Controller Theta : Subsystem
  PIDF Controller theta Kd 2D Lookup Table : Lookup_n-D  BreakpointsForDimension1=SkywalkerX8.Control.Longitudinal.SchedulingVariables.VaArray  BreakpointsForDimension2=SkywalkerX8.Control.Longitudinal.SchedulingVariables.alphaArray  Table=SkywalkerX8.Control.Longitudinal.thetaController.KdTheta  InternalRulePriority=Speed  RndMeth=Simplest  InputSameDT=on
  PIDF Controller theta Ki 2D Lookup Table : Lookup_n-D  BreakpointsForDimension1=SkywalkerX8.Control.Longitudinal.SchedulingVariables.VaArray  BreakpointsForDimension2=SkywalkerX8.Control.Longitudinal.SchedulingVariables.alphaArray  Table=SkywalkerX8.Control.Longitudinal.thetaController.KiTheta  InternalRulePriority=Speed  RndMeth=Simplest  InputSameDT=on
  PIDF Controller theta Kp 2D Lookup Table : Lookup_n-D  BreakpointsForDimension1=SkywalkerX8.Control.Longitudinal.SchedulingVariables.VaArray  BreakpointsForDimension2=SkywalkerX8.Control.Longitudinal.SchedulingVariables.alphaArray  Table=SkywalkerX8.Control.Longitudinal.thetaController.KpTheta  InternalRulePriority=Speed  RndMeth=Simplest  InputSameDT=on
  PIDF Controller theta N 2D Lookup Table : Lookup_n-D  BreakpointsForDimension1=SkywalkerX8.Control.Longitudinal.SchedulingVariables.VaArray  BreakpointsForDimension2=SkywalkerX8.Control.Longitudinal.SchedulingVariables.alphaArray  Table=SkywalkerX8.Control.Longitudinal.thetaController.NTheta  InternalRulePriority=Speed  RndMeth=Simplest  InputSameDT=on
  Saturation : Saturate  UpperLimit=SkywalkerX8.Control.Longitudinal.thetaController.upperSaturationNegativeDe  LowerLimit=SkywalkerX8.Control.Longitudinal.thetaController.lowerSaturationNegativeDe
  Sign Inversion : Gain  Gain=-1
  Sum1 : Sum  Inputs=+++|
  de : Outport
  wires:
  Va/1 -> PDF Controller theta 2DOF Kd 2D Lookup Table/1, PDF Controller theta 2DOF Kp 2D Lookup Table/1, PDF Controller theta 2DOF N 2D Lookup Table/1, PIDF Controller theta N 2D Lookup Table/1, PIDF Controller theta Kd 2D Lookup Table/1, PIDF Controller theta Ki 2D Lookup Table/1, PIDF Controller theta Kp 2D Lookup Table/1
  theta_e/1 -> PI Controller Theta/1(u)
  PIDF Controller theta Kp 2D Lookup Table/1 -> PI Controller Theta/2(P)
  PIDF Controller theta Ki 2D Lookup Table/1 -> PI Controller Theta/3(I)
  alpha/1 -> PDF Controller theta 2DOF N 2D Lookup Table/2, PDF Controller theta 2DOF Kd 2D Lookup Table/2, PDF Controller theta 2DOF Kp 2D Lookup Table/2, PIDF Controller theta N 2D Lookup Table/2, PIDF Controller theta Kd 2D Lookup Table/2, PIDF Controller theta Ki 2D Lookup Table/2, PIDF Controller theta Kp 2D Lookup Table/2
  PI Controller Theta/1(y) -> Sum1/2
  Sum1/1 -> Saturation/1, PI Controller Theta/5(Pre-Saturation)
  Saturation/1 -> Sign Inversion/1, PI Controller Theta/4(Post-Saturation)
  PIDF Controller theta N 2D Lookup Table/1 -> DF Controller Theta/1(N)
  PIDF Controller theta Kd 2D Lookup Table/1 -> DF Controller Theta/2(D)
  q/1 -> DF Controller Theta/3(du/dt)
  DF Controller Theta/1(de*) -> Sum1/3
  Sign Inversion/1 -> de/1
  PDF Controller theta 2DOF Kp 2D Lookup Table/1 -> PDF Controller Theta 2DOF/2(P)
  PDF Controller theta 2DOF Kd 2D Lookup Table/1 -> PDF Controller Theta 2DOF/3(D)
  PDF Controller theta 2DOF N 2D Lookup Table/1 -> PDF Controller Theta 2DOF/4(N)
  Ref/1 -> PDF Controller Theta 2DOF/1(u)
  PDF Controller Theta 2DOF/1(y) -> Sum1/1

== system SkywalkerX8_Control/Autopilot/Gain Scheduled Controller Va_dt ==
  Va_e : Inport
  Va : Inport  Port=2
  TR : Inport  Port=3
  PIDF Controller Va_dt : Subsystem
  PIDF Controller Va_dt Kd 2D Lookup Table : Lookup_n-D  NumberOfTableDimensions=1  BreakpointsForDimension1=SkywalkerX8.Control.Longitudinal.SchedulingVariables.VaArray  BreakpointsForDimension2=[1 2 3 4 5]  Table=SkywalkerX8.Control.Longitudinal.VaDtController.KdVaDt  InternalRulePriority=Speed  RndMeth=Simplest  InputSameDT=on
  PIDF Controller Va_dt Ki 2D Lookup Table : Lookup_n-D  NumberOfTableDimensions=1  BreakpointsForDimension1=SkywalkerX8.Control.Longitudinal.SchedulingVariables.VaArray  BreakpointsForDimension2=[1 2 3 4 5]  Table=SkywalkerX8.Control.Longitudinal.VaDtController.KiVaDt  InternalRulePriority=Speed  RndMeth=Simplest  InputSameDT=on
  PIDF Controller Va_dt Kp 2D Lookup Table : Lookup_n-D  NumberOfTableDimensions=1  BreakpointsForDimension1=SkywalkerX8.Control.Longitudinal.SchedulingVariables.VaArray  BreakpointsForDimension2=[1 2 3 4 5]  Table=SkywalkerX8.Control.Longitudinal.VaDtController.KpVaDt  InternalRulePriority=Speed  RndMeth=Simplest  InputSameDT=on
  PIDF Controller Va_dt Kt Tracking Gain Scalar : Gain  Gain=SkywalkerX8.Control.Longitudinal.VaDtController.KtScalar
  PIDF Controller Va_dt N 2D Lookup Table : Lookup_n-D  NumberOfTableDimensions=1  BreakpointsForDimension1=SkywalkerX8.Control.Longitudinal.SchedulingVariables.VaArray  BreakpointsForDimension2=[1 2 3 4 5]  Table=SkywalkerX8.Control.Longitudinal.VaDtController.NVaDt  InternalRulePriority=Speed  RndMeth=Simplest  InputSameDT=on
  dt : Outport
  wires:
  Va_e/1 -> PIDF Controller Va_dt/1(u)
  PIDF Controller Va_dt/1(y) -> dt/1
  PIDF Controller Va_dt Kp 2D Lookup Table/1 -> PIDF Controller Va_dt/2(P)
  Va/1 -> PIDF Controller Va_dt N 2D Lookup Table/1, PIDF Controller Va_dt Kd 2D Lookup Table/1, PIDF Controller Va_dt Ki 2D Lookup Table/1, PIDF Controller Va_dt Kp 2D Lookup Table/1
  PIDF Controller Va_dt Ki 2D Lookup Table/1 -> PIDF Controller Va_dt/3(I), PIDF Controller Va_dt Kt Tracking Gain Scalar/1
  PIDF Controller Va_dt Kd 2D Lookup Table/1 -> PIDF Controller Va_dt/4(D)
  PIDF Controller Va_dt N 2D Lookup Table/1 -> PIDF Controller Va_dt/5(N)
  TR/1 -> PIDF Controller Va_dt/7(TR)
  PIDF Controller Va_dt Kt Tracking Gain Scalar/1 -> PIDF Controller Va_dt/6(Kt)

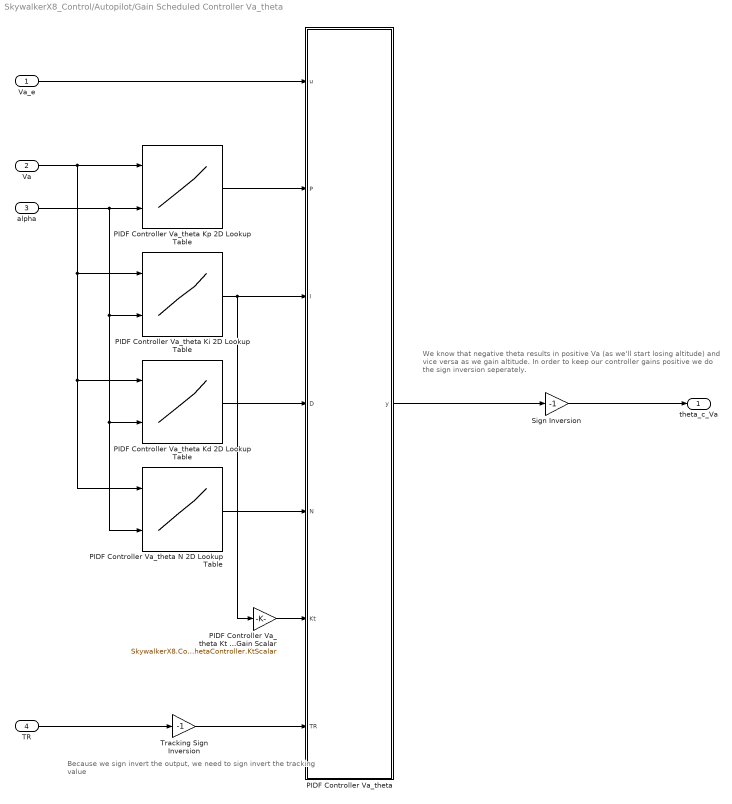
== system SkywalkerX8_Control/Autopilot/Gain Scheduled Controller Va_theta ==
  note: We know that negative theta results in positive Va (as we'll start losing altitude)
      | and vice versa as we gain altitude. In order to keep our controller gains positive
      |  we do the sign inversion seperately.
  note: Because we sign invert the output, we need to sign invert the tracking
      | value
  Va_e : Inport
  Va : Inport  Port=2
  alpha : Inport  Port=3
  TR : Inport  Port=4
  PIDF Controller Va_theta : Subsystem
  PIDF Controller Va_theta Kd 2D Lookup Table : Lookup_n-D  BreakpointsForDimension1=SkywalkerX8.Control.Longitudinal.SchedulingVariables.VaArray  BreakpointsForDimension2=SkywalkerX8.Control.Longitudinal.SchedulingVariables.alphaArray  Table=SkywalkerX8.Control.Longitudinal.VaThetaController.KdVaTheta  InternalRulePriority=Speed  RndMeth=Simplest  InputSameDT=on
  PIDF Controller Va_theta Ki 2D Lookup Table : Lookup_n-D  BreakpointsForDimension1=SkywalkerX8.Control.Longitudinal.SchedulingVariables.VaArray  BreakpointsForDimension2=SkywalkerX8.Control.Longitudinal.SchedulingVariables.alphaArray  Table=SkywalkerX8.Control.Longitudinal.VaThetaController.KiVaTheta  InternalRulePriority=Speed  RndMeth=Simplest  InputSameDT=on
  PIDF Controller Va_theta Kp 2D Lookup Table : Lookup_n-D  BreakpointsForDimension1=SkywalkerX8.Control.Longitudinal.SchedulingVariables.VaArray  BreakpointsForDimension2=SkywalkerX8.Control.Longitudinal.SchedulingVariables.alphaArray  Table=SkywalkerX8.Control.Longitudinal.VaThetaController.KpVaTheta  InternalRulePriority=Speed  RndMeth=Simplest  InputSameDT=on
  PIDF Controller Va_theta Kt Tracking Gain Scalar : Gain  Gain=SkywalkerX8.Control.Longitudinal.VaThetaController.KtScalar
  PIDF Controller Va_theta N 2D Lookup Table : Lookup_n-D  BreakpointsForDimension1=SkywalkerX8.Control.Longitudinal.SchedulingVariables.VaArray  BreakpointsForDimension2=SkywalkerX8.Control.Longitudinal.SchedulingVariables.alphaArray  Table=SkywalkerX8.Control.Longitudinal.VaThetaController.NVaTheta  InternalRulePriority=Speed  RndMeth=Simplest  InputSameDT=on
  Sign Inversion : Gain  Gain=-1
  Tracking Sign Inversion : Gain  Gain=-1
  theta_c_Va : Outport
  wires:
  Va_e/1 -> PIDF Controller Va_theta/1(u)
  PIDF Controller Va_theta/1(y) -> Sign Inversion/1
  PIDF Controller Va_theta Kp 2D Lookup Table/1 -> PIDF Controller Va_theta/2(P)
  Va/1 -> PIDF Controller Va_theta Kd 2D Lookup Table/1, PIDF Controller Va_theta N 2D Lookup Table/1, PIDF Controller Va_theta Ki 2D Lookup Table/1, PIDF Controller Va_theta Kp 2D Lookup Table/1
  PIDF Controller Va_theta Ki 2D Lookup Table/1 -> PIDF Controller Va_theta Kt Tracking Gain Scalar/1, PIDF Controller Va_theta/3(I)
  PIDF Controller Va_theta Kd 2D Lookup Table/1 -> PIDF Controller Va_theta/4(D)
  PIDF Controller Va_theta N 2D Lookup Table/1 -> PIDF Controller Va_theta/5(N)
  alpha/1 -> PIDF Controller Va_theta N 2D Lookup Table/2, PIDF Controller Va_theta Kd 2D Lookup Table/2, PIDF Controller Va_theta Ki 2D Lookup Table/2, PIDF Controller Va_theta Kp 2D Lookup Table/2
  Sign Inversion/1 -> theta_c_Va/1
  TR/1 -> Tracking Sign Inversion/1
  PIDF Controller Va_theta Kt Tracking Gain Scalar/1 -> PIDF Controller Va_theta/6(Kt)
  Tracking Sign Inversion/1 -> PIDF Controller Va_theta/7(TR)

== system SkywalkerX8_Control/Autopilot/Gain Scheduled Controller h_theta ==
  note: We know that wings-level trim has the aircraft with a pitch angle. As such,
      | we know that at a minimum this controller has to be a PI controller, because otherwise
      | we have no state to hold the required steady state theta command.
  h_e : Inport
  Va : Inport  Port=2
  alpha : Inport  Port=3
  TR : Inport  Port=4
  PIDF Controller h_theta : Subsystem
  PIDF Controller h_theta Kd 2D Lookup Table : Lookup_n-D  BreakpointsForDimension1=SkywalkerX8.Control.Longitudinal.SchedulingVariables.VaArray  BreakpointsForDimension2=SkywalkerX8.Control.Longitudinal.SchedulingVariables.alphaArray  Table=SkywalkerX8.Control.Longitudinal.altController.KdAlt  InternalRulePriority=Speed  RndMeth=Simplest  InputSameDT=on
  PIDF Controller h_theta Ki 2D Lookup Table : Lookup_n-D  BreakpointsForDimension1=SkywalkerX8.Control.Longitudinal.SchedulingVariables.VaArray  BreakpointsForDimension2=SkywalkerX8.Control.Longitudinal.SchedulingVariables.alphaArray  Table=SkywalkerX8.Control.Longitudinal.altController.KiAlt  InternalRulePriority=Speed  RndMeth=Simplest  InputSameDT=on
  PIDF Controller h_theta Kp 2D Lookup Table : Lookup_n-D  BreakpointsForDimension1=SkywalkerX8.Control.Longitudinal.SchedulingVariables.VaArray  BreakpointsForDimension2=SkywalkerX8.Control.Longitudinal.SchedulingVariables.alphaArray  Table=SkywalkerX8.Control.Longitudinal.altController.KpAlt  InternalRulePriority=Speed  RndMeth=Simplest  InputSameDT=on
  PIDF Controller h_theta Kt Tracking Gain Scalar : Gain  Gain=SkywalkerX8.Control.Longitudinal.altController.KtScalar
  PIDF Controller h_theta N 2D Lookup Table : Lookup_n-D  BreakpointsForDimension1=SkywalkerX8.Control.Longitudinal.SchedulingVariables.VaArray  BreakpointsForDimension2=SkywalkerX8.Control.Longitudinal.SchedulingVariables.alphaArray  Table=SkywalkerX8.Control.Longitudinal.altController.NAlt  InternalRulePriority=Speed  RndMeth=Simplest  InputSameDT=on
  theta_c_h : Outport
  wires:
  PIDF Controller h_theta Kp 2D Lookup Table/1 -> PIDF Controller h_theta/2(P)
  alpha/1 -> PIDF Controller h_theta Ki 2D Lookup Table/2, PIDF Controller h_theta N 2D Lookup Table/2, PIDF Controller h_theta Kd 2D Lookup Table/2, PIDF Controller h_theta Kp 2D Lookup Table/2
  h_e/1 -> PIDF Controller h_theta/1(u)
  Va/1 -> PIDF Controller h_theta Ki 2D Lookup Table/1, PIDF Controller h_theta N 2D Lookup Table/1, PIDF Controller h_theta Kd 2D Lookup Table/1, PIDF Controller h_theta Kp 2D Lookup Table/1
  PIDF Controller h_theta Kd 2D Lookup Table/1 -> PIDF Controller h_theta/4(D)
  PIDF Controller h_theta N 2D Lookup Table/1 -> PIDF Controller h_theta/5(N)
  PIDF Controller h_theta/1(y) -> theta_c_h/1
  TR/1 -> PIDF Controller h_theta/7(TR)
  PIDF Controller h_theta Ki 2D Lookup Table/1 -> PIDF Controller h_theta Kt Tracking Gain Scalar/1, PIDF Controller h_theta/3(I)
  PIDF Controller h_theta Kt Tracking Gain Scalar/1 -> PIDF Controller h_theta/6(Kt)

== system SkywalkerX8_Control/Autopilot/Va Rate Limiter ==
  note: U(k)
  note: Y(k)
  up : Inport
  u : Inport  Port=2
  lo : Inport  Port=3
  Delay Input2 : UnitDelay  Description=Store in Global RAM  DisableCoverage=on  InitialCondition=initOutput  SampleTime=-1
  Difference Inputs1 : Sum  Description=Add in CPU  DisableCoverage=on  Inputs=+-  OutDataTypeStr=Inherit: Inherit via back propagation
  Difference Inputs2 : Sum  Description=Add in CPU  OutDataTypeStr=Inherit: Inherit via back propagation
  FixPt Data Type Duplicate : DataTypeDuplicate  DisableCoverage=on  NumInputPorts=7
  Saturation Dynamic : simulink/Discontinuities/Saturation Dynamic  OutMin=[]  OutMax=[]  OutDataTypeStr=Inherit: Same as second input  OutDataType=fixdt(1, 16)  OutScaling=2^-10  DoSatur=off
  delta fall limit : Product  DisableCoverage=on  Inputs=**  OutDataTypeStr=Inherit: Inherit via back propagation  SaturateOnIntegerOverflow=on
  delta rise limit : Product  DisableCoverage=on  Inputs=**  OutDataTypeStr=Inherit: Inherit via back propagation  SaturateOnIntegerOverflow=on
  sample time : SampleTimeMath  DisableCoverage=on  TsampMathOp=Ts Only  weightValue=1
  Y : Outport  InitialOutput=0
  wires:
  Delay Input2/1 -> Difference Inputs1/2, FixPt Data Type Duplicate/2, Difference Inputs2/2  "Y(k-1)"
  Difference Inputs1/1 -> FixPt Data Type Duplicate/4, Saturation Dynamic/2  "( U(k) - Y(k-1) )"
  Difference Inputs2/1 -> Y/1, Delay Input2/1, FixPt Data Type Duplicate/1
  u/1 -> Difference Inputs1/1, FixPt Data Type Duplicate/5, sample time/1
  delta fall limit/1 -> FixPt Data Type Duplicate/3, Saturation Dynamic/3
  sample time/1 -> delta fall limit/2, delta rise limit/2
  Saturation Dynamic/1 -> Difference Inputs2/1, FixPt Data Type Duplicate/7
  delta rise limit/1 -> FixPt Data Type Duplicate/6, Saturation Dynamic/1
  lo/1 -> delta fall limit/1
  up/1 -> delta rise limit/1

== system SkywalkerX8_Control/Autopilot/h Rate Limiter Dynamic ==
  note: U(k)
  note: Y(k)
  up : Inport
  u : Inport  Port=2
  lo : Inport  Port=3
  Delay Input2 : UnitDelay  Description=Store in Global RAM  DisableCoverage=on  InitialCondition=initOutput  SampleTime=-1
  Difference Inputs1 : Sum  Description=Add in CPU  DisableCoverage=on  Inputs=+-  OutDataTypeStr=Inherit: Inherit via back propagation
  Difference Inputs2 : Sum  Description=Add in CPU  OutDataTypeStr=Inherit: Inherit via back propagation
  FixPt Data Type Duplicate : DataTypeDuplicate  DisableCoverage=on  NumInputPorts=7
  Saturation Dynamic : simulink/Discontinuities/Saturation Dynamic  OutMin=[]  OutMax=[]  OutDataTypeStr=Inherit: Same as second input  OutDataType=fixdt(1, 16)  OutScaling=2^-10  DoSatur=off
  delta fall limit : Product  DisableCoverage=on  Inputs=**  OutDataTypeStr=Inherit: Inherit via back propagation  SaturateOnIntegerOverflow=on
  delta rise limit : Product  DisableCoverage=on  Inputs=**  OutDataTypeStr=Inherit: Inherit via back propagation  SaturateOnIntegerOverflow=on
  sample time : SampleTimeMath  DisableCoverage=on  TsampMathOp=Ts Only  weightValue=1
  Y : Outport  InitialOutput=0
  wires:
  Delay Input2/1 -> Difference Inputs1/2, FixPt Data Type Duplicate/2, Difference Inputs2/2  "Y(k-1)"
  Difference Inputs1/1 -> FixPt Data Type Duplicate/4, Saturation Dynamic/2  "( U(k) - Y(k-1) )"
  Difference Inputs2/1 -> Y/1, Delay Input2/1, FixPt Data Type Duplicate/1
  u/1 -> Difference Inputs1/1, FixPt Data Type Duplicate/5, sample time/1
  delta fall limit/1 -> FixPt Data Type Duplicate/3, Saturation Dynamic/3
  sample time/1 -> delta fall limit/2, delta rise limit/2
  Saturation Dynamic/1 -> Difference Inputs2/1, FixPt Data Type Duplicate/7
  delta rise limit/1 -> FixPt Data Type Duplicate/6, Saturation Dynamic/1
  lo/1 -> delta fall limit/1
  up/1 -> delta rise limit/1

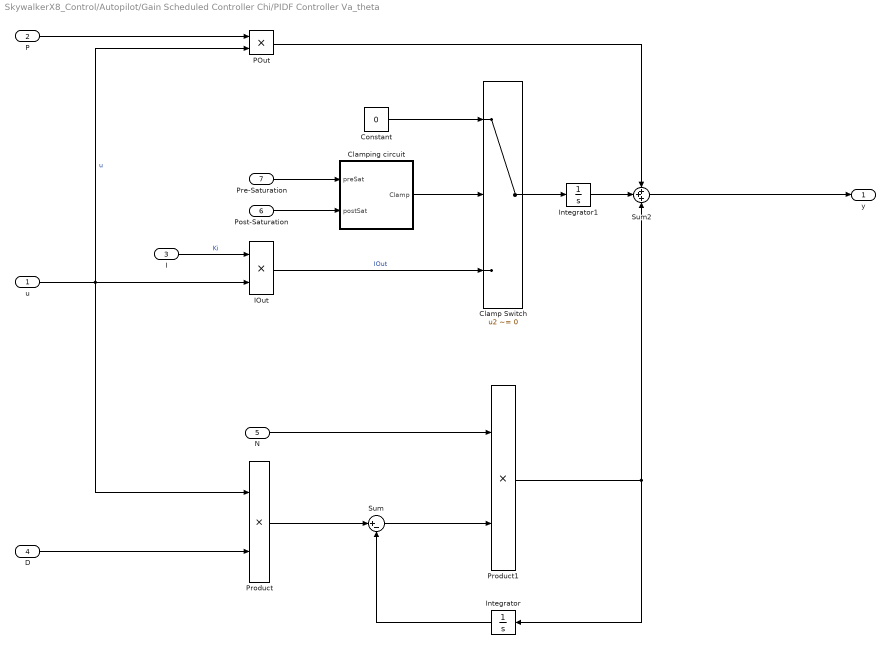
== system SkywalkerX8_Control/Autopilot/Gain Scheduled Controller Chi/PIDF Controller Va_theta ==
  u : Inport
  P : Inport  Port=2
  I : Inport  Port=3
  D : Inport  Port=4
  N : Inport  Port=5
  Post-Saturation : Inport  Port=6
  Pre-Saturation : Inport  Port=7
  Clamp Switch : Switch  Criteria=u2 ~= 0
  Clamping circuit : Subsystem
  Constant : Constant  Value=0
  IOut : Product  DisableCoverage=on
  Integrator : Integrator
  Integrator1 : Integrator  IgnoreLimit=on
  POut : Product
  Product : Product
  Product1 : Product
  Sum : Sum  Inputs=|+-
  Sum2 : Sum  Inputs=+++
  y : Outport  InitialOutput=0
  wires:
  Sum2/1 -> y/1
  N/1 -> Product1/1
  Product1/1 -> Sum2/3, Integrator/1
  Sum/1 -> Product1/2
  POut/1 -> Sum2/1
  D/1 -> Product/2
  u/1 -> POut/2, Product/1, IOut/2  "u"
  Integrator/1 -> Sum/2
  Clamp Switch/1 -> Integrator1/1
  Product/1 -> Sum/1
  Integrator1/1 -> Sum2/2
  Constant/1 -> Clamp Switch/1
  I/1 -> IOut/1  "Ki"
  IOut/1 -> Clamp Switch/3  "IOut"
  Clamping circuit/1(Clamp) -> Clamp Switch/2
  P/1 -> POut/1
  Pre-Saturation/1 -> Clamping circuit/1(preSat)
  Post-Saturation/1 -> Clamping circuit/2(postSat)

== system SkywalkerX8_Control/Autopilot/Gain Scheduled Controller Phi/DF Controller Phi ==
  N : Inport
  D : Inport  Port=2
  du/dt : Inport  Port=3
  Integrator : Integrator
  Product : Product
  Product1 : Product
  Sum : Sum  Inputs=|+-
  da* : Outport
  wires:
  Integrator/1 -> da*/1, Sum/2  "da*"
  Product1/1 -> Integrator/1  "Nda*_e"
  du/dt/1 -> Product/2
  D/1 -> Product/1
  Sum/1 -> Product1/2  "da*_e"
  N/1 -> Product1/1
  Product/1 -> Sum/1
